simulink model "dynsim_test_urdf"  (R2020a)
settings: Solver=FixedStepAuto  StartTime=0.0  StopTime=6  FixedStep=0.001  RelTol=1e-3
libraries: robotmaniplib x2
settings Model: SimulationMode=accelerator  Creator=bascetta  LastModifiedBy=alberto
settings OptimizationCC: EnhancedBackFolding=on  PassReuseOutputArgsAs=Individual arguments  ZeroExternalMemoryAtStartup=off  ZeroInternalMemoryAtStartup=off  MaxStackSize=64  OptimizeBlockOrder=speed  DifferentSizesBufferReuse=on  OptimizationCustomize=off  EfficientTunableParamExpr=on
settings DebuggingCC: ParameterTunabilityLossMsg=error
settings HardwareCC: ProdBitPerPointer=32  ProdBitPerSizeT=32  ProdBitPerPtrDiffT=32  ProdLargestAtomicFloat=None  ProdIntDivRoundTo=Undefined  ProdEndianess=Unspecified  ProdWordSize=32  ProdHWDeviceType=Generic->Unspecified (assume 32-bit Generic)
settings RTWCC: SystemTargetFile=ert.tlc  HardwareBoard=Robot Operating System (ROS)  TemplateMakefile=ert_default_tmf  GenerateReport=on  Toolchain=Catkin  IncludeHyperlinkInReport=on  LaunchReport=on  TargetLang=C++  GenerateTraceInfo=on  GenerateTraceReport=on  GenerateTraceReportSl=on  GenerateTraceReportSf=on  GenerateTraceReportEml=on
settings CodeAppCC: ForceParamTrailComments=on  IgnoreCustomStorageClasses=off  OperatorAnnotations=on  SimulinkDataObjDesc=on  SFDataObjDesc=on  InsertBlockDesc=on
settings ERTTargetCC: SupportContinuousTime=on  SupportVariableSizeSignals=on

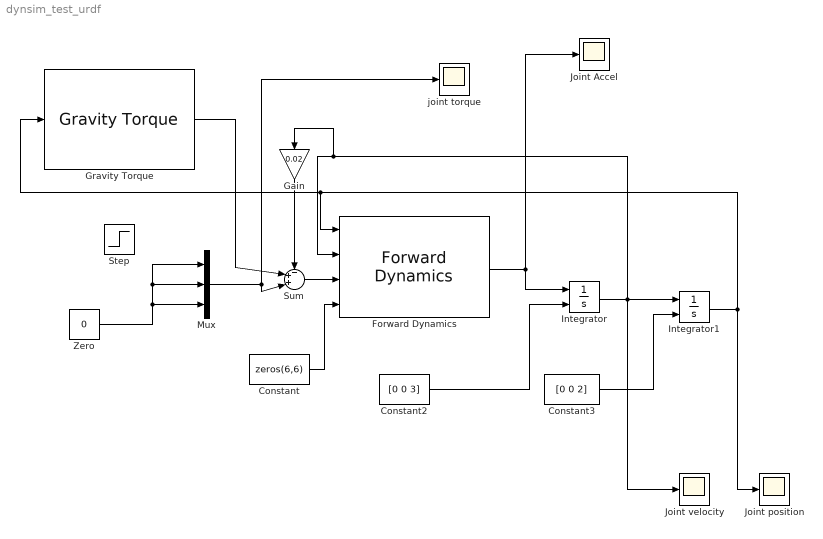
== system dynsim_test_urdf ==
  Constant : Constant  Value=zeros(6,6)
  Constant2 : Constant  Value=[0 0 3]
  Constant3 : Constant  Value=[0 0 2]
  Forward Dynamics : robotmaniplib/Forward Dynamics  RigidBodyTree=robot_edo_nuove_inerzie  SimulateUsing=Interpreted execution
  Gain : Gain  Gain=0.02
  Gravity Torque : robotmaniplib/Gravity Torque  RigidBodyTree=robot_edo_nuove_inerzie  SimulateUsing=Interpreted execution
  Integrator : Integrator  InitialConditionSource=external
  Integrator1 : Integrator  InitialConditionSource=external
  Joint Accel : Scope
  Joint position : Scope
  Joint velocity : Scope
  Mux : Mux  Inputs=3
  Step : Step  After=0.2  SampleTime=0
  Sum : Sum  Inputs=-++|
  Zero : Constant  Value=0  OutDataTypeStr=Inherit: Inherit via back propagation
  joint torque : Scope
  wires:
  Constant/1 -> Forward Dynamics/4
  Forward Dynamics/1 -> Integrator/1, Joint Accel/1
  Integrator1/1 -> Gravity Torque/1, Forward Dynamics/1, Joint position/1
  Constant2/1 -> Integrator/2
  Constant3/1 -> Integrator1/2
  Integrator/1 -> Joint velocity/1, Gain/1, Forward Dynamics/2, Integrator1/1
  Mux/1 -> Sum/3, joint torque/1
  Zero/1 -> Mux/3, Mux/1, Mux/2
  Sum/1 -> Forward Dynamics/3
  Gain/1 -> Sum/1
  Gravity Torque/1 -> Sum/2
